simulink model "model_based"  (R2019a)
settings: Solver=VariableStepAuto  StartTime=0.0  StopTime=10.0  RelTol=1e-3
values from neighbouring files (symbols this model uses):
  J = 1    [dc_motor_simulink_modelling.m]
  K = 1    [dc_motor_simulink_modelling.m]
  L = 1    [dc_motor_simulink_modelling.m]
  R = 1    [dc_motor_simulink_modelling.m]
settings Model: Creator=fotoyis  LastModifiedBy=fotoyis

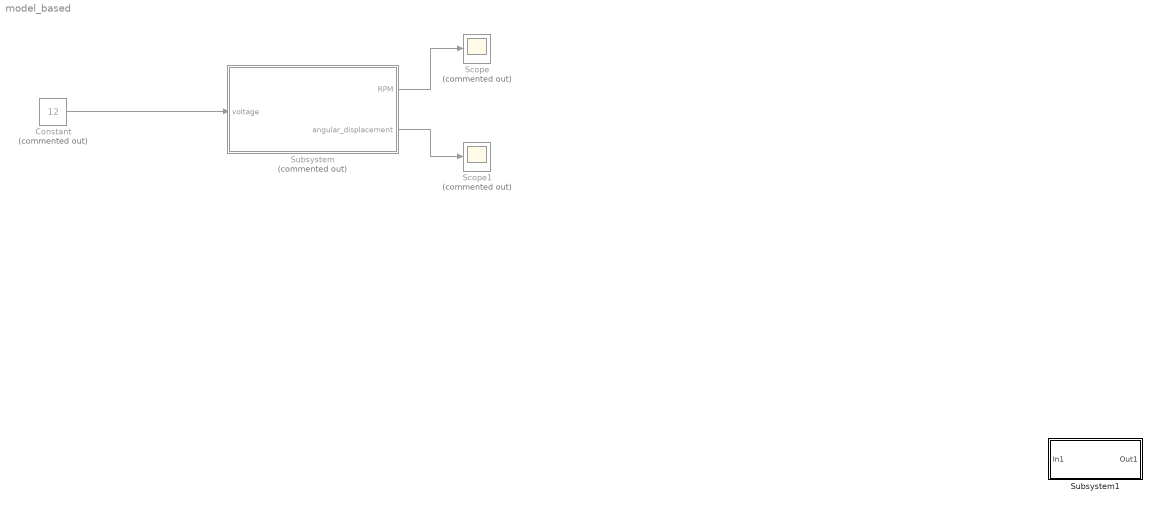
== system model_based ==
  Constant : Constant  Commented=on  Value=12
  Scope : Scope  Commented=on
  Scope1 : Scope  Commented=on
  Subsystem : Subsystem  Commented=on
  Subsystem1 : Subsystem
  wires:
  Constant/1 -> Subsystem/1(voltage)
  Subsystem/1(RPM) -> Scope/1
  Subsystem/2(angular_displacement) -> Scope1/1

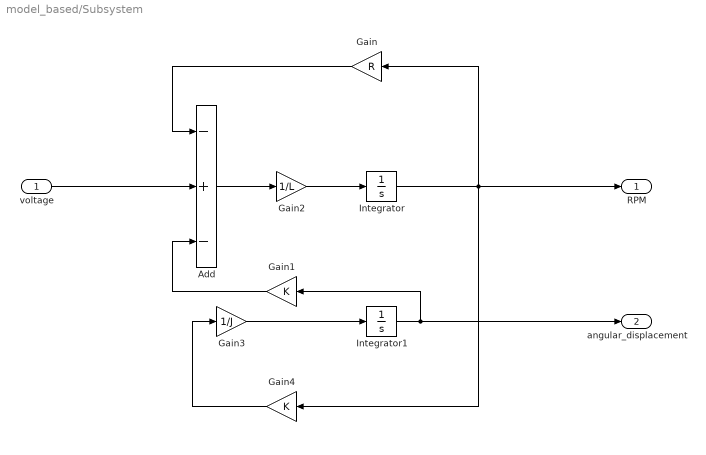
== system model_based/Subsystem ==
  voltage : Inport
  Add : Sum  Inputs=-+-
  Gain : Gain  Gain=R
  Gain1 : Gain  Gain=K
  Gain2 : Gain  Gain=1/L
  Gain3 : Gain  Gain=1/J
  Gain4 : Gain  Gain=K
  Integrator : Integrator
  Integrator1 : Integrator
  RPM : Outport
  angular_displacement : Outport  Port=2
  wires:
  Integrator/1 -> RPM/1, Gain4/1, Gain/1
  Integrator1/1 -> angular_displacement/1, Gain1/1
  Gain2/1 -> Integrator/1
  Gain/1 -> Add/1
  Add/1 -> Gain2/1
  voltage/1 -> Add/2
  Gain4/1 -> Gain3/1
  Gain1/1 -> Add/3
  Gain3/1 -> Integrator1/1

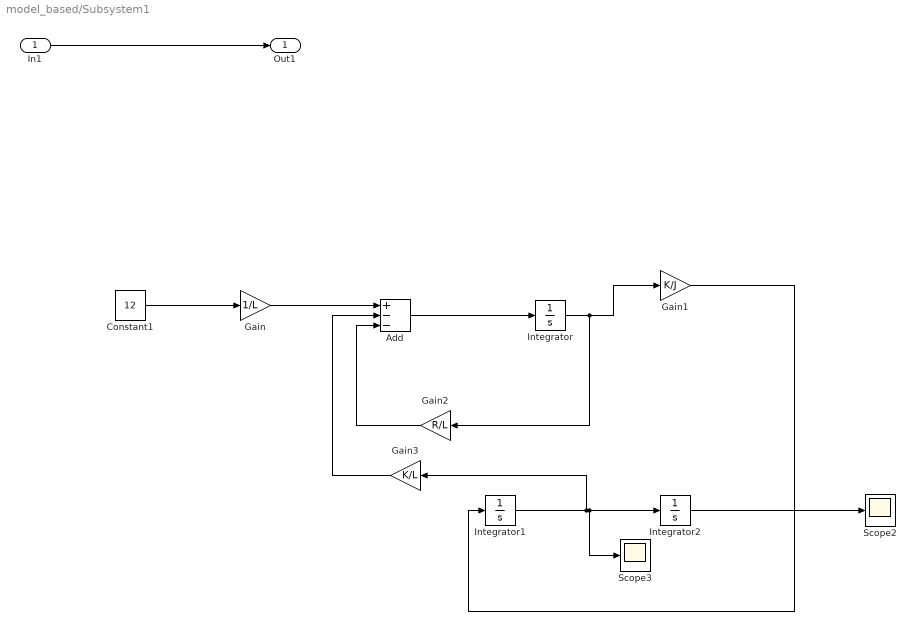
== system model_based/Subsystem1 ==
  In1 : Inport
  Add : Sum  Inputs=+--
  Constant1 : Constant  Value=12
  Gain : Gain  Gain=1/L
  Gain1 : Gain  Gain=K/J
  Gain2 : Gain  Gain=R/L
  Gain3 : Gain  Gain=K/L
  Integrator : Integrator
  Integrator1 : Integrator
  Integrator2 : Integrator
  Scope2 : Scope
  Scope3 : Scope
  Out1 : Outport
  wires:
  In1/1 -> Out1/1
  Integrator/1 -> Gain2/1, Gain1/1
  Integrator2/1 -> Scope2/1
  Constant1/1 -> Gain/1
  Gain3/1 -> Add/2
  Gain2/1 -> Add/3
  Gain/1 -> Add/1
  Add/1 -> Integrator/1
  Integrator1/1 -> Gain3/1, Scope3/1, Integrator2/1
  Gain1/1 -> Integrator1/1
